simulink model "tasks_union_2"  (R2020b)
settings: Solver=FixedStepAuto  StartTime=0.0  StopTime=5  FixedStep=0.001  RelTol=1e-3
values from neighbouring files (symbols this model uses):
  a = evalin('base','a')    [Coriolis.m]    (also in init.m = 0.5)
  a0 = 0.99    [init.m]
  ac = mass_can*(l1*l2)    (= 0.5)    [init.m]
  berta = 0.98    [init.m]
  csi = 1    [init.m]
  D_high = [sqrt(4*M*K_high(1,1)) 0; 0 sqrt(4*M*K_high(2,2))]    [init.m]
  D_low = [sqrt(4*M*K_low(1,1)) 0; 0 sqrt(4*M*K_low(2,2))]    [init.m]
  e_max = 0.01    [init.m]
  F_int_max = [2;2]    [init.m]
  F_max = [2;2]    [init.m]
  g = evalin('base','g')    [Gravity.m]    (also in init.m = 9.81)
  I1 = evalin('base','I1')    [Mass.m]    (also in init.m = 1)
  I2 = evalin('base','I2')    [Mass.m]    (also in init.m = 1)
  Ic = mass_can*l2^2    (= 0.5)    [init.m]
  K_high = [F_max(1)/e_max 0; 0 (mass_can*g)/e_max]    [init.m]
  K_low = [20 0; 0 20]    [init.m]
  l1 = evalin('base','l1')    [Gravity.m]    (also in Jacobianoa_dot.m; Mass.m; cin_dir.m; init.m = 1)
  l2 = evalin('base','l2')    [Gravity.m]    (also in Jacobianoa_dot.m; Mass.m; cin_dir.m; init.m = 1)
  M = 0.1    [init.m]
  m1 = evalin('base','m1')    [Gravity.m]    (also in Mass.m; init.m = 1)
  m2 = evalin('base','m2')    [Gravity.m]    (also in Mass.m; init.m = 1)
  mass = 0.1    [init.m]
  mass_can = 0.5    [init.m]
libraries: simulink x1
(part 2 of 2)

== matlab function tasks_union_2/RR_Model_Joint_Space/MASS^-1 ==
  data: q input size=2; ddq output size=2; F_tot input double size=2; I1 parameter; I2 parameter; l1 parameter; l2 parameter; m1 parameter; m2 parameter; grasping input; Ic parameter; mass_can parameter
function ddq = fcn(q,F_tot,I1, I2, l1, l2, m1, m2, grasping, Ic, mass_can)

mc = mass_can;

B = [((l1^2)/4)*m1 + I1 + m2*(l1^2) + m2*((l2^2)/4) + m2*l1*l2*cos(q(2)) + I2, m2*(((l1*l2)/2)*cos(q(2)) + (l2^2)/4) + I2; ...
    m2*(((l1*l2)/2)*cos(q(2)) + (l2^2)/4) + I2, m2*(l2^2)/4 + I2];

% if grasping == 1
%     Bc = [mc*((l1^2) + (l2^2) +2*l1*l2*cos(q(2))) + Ic, mc*((l2^2) + l1*l2*cos(q(2))) + Ic; ...
%           mc*((l2^2) + l1*l2*cos(q(2))) + Ic, mc*(l2^2)+ Ic];
%     B = B + Bc;
% end

ddq = B\F_tot;                      % Ftot*M^-1

end

== matlab function tasks_union_2/RR_Model_Joint_Space/MATLAB Function ==
  data: F input size=2; F_ext output double size=2; q input size=2; l1 parameter; l2 parameter
function F_ext = fcn(F,q,l1, l2)


Ja = [-l1*sin(q(1)) - l2*sin(q(1)+q(2)), -l2*sin(q(1)+q(2)); ...
    l1*cos(q(1)) + l2*cos(q(1)+q(2)), l2*cos(q(1)+q(2))];

F_ext = Ja'*F;

end

== matlab function tasks_union_2/Dyrect Kinematics ==
  data: q_dot input double size=2; dz output double size=2; q input double size=2; z output double size=2; l1 parameter; l2 parameter
function [dz,z] = fcn(q_dot,q,l1, l2)

z = zeros(2,1);
z(1) = l1*cos(q(1)) + l2*cos(q(1)+q(2));
z(2) = l1*sin(q(1)) + l2*sin(q(1)+q(2));

Ja = zeros(2,2);
Ja = [-l1*sin(q(1)) - l2*sin(q(1)+q(2)), -l2*sin(q(1)+q(2)); ...
    l1*cos(q(1)) + l2*cos(q(1)+q(2)), l2*cos(q(1)+q(2))];

dz = zeros(2,1);
dz = Ja*q_dot;

end

== matlab function tasks_union_2/PLANNER3/INTERPOLATOR OF K AND D  ==
  settings: updateMethod=DISCRETE
  data: time input; K output; kx_f input; ky_f input; D output; e_max parameter; F_max parameter; M parameter; berta parameter; a0 parameter; mass parameter; csi parameter
function [K,D] = fcn(time, kx_f, ky_f, e_max, F_max,M, berta, a0, mass, csi)

persistent kx ky time_prec

if isempty(time_prec)
    time_prec = 0;
end

if isempty(kx)
   kx = F_max(1)/e_max; 
end
if isempty(ky)
   ky = F_max(2)/e_max;
end

% everytime k is increasing in accordance with stability condition
if kx_f <= kx
    kx = kx_f;
else 
    kx_i = kx;
    k_dotx = berta*(4*a0*sqrt(kx_i/mass)*(kx_i)^(3/2))/(sqrt(kx_i) + 2*a0*csi*sqrt(kx_i));
    k_tempx = kx_i + k_dotx*(time -time_prec);
    if k_tempx > kx_f
        kx = kx_f;
    else
        kx = k_tempx;
    end
end

if ky_f <= ky
    ky = ky_f;
else 
    ky_i = ky;
    k_doty = berta*(4*a0*sqrt(ky_i/mass)*(ky_i)^(3/2))/(sqrt(ky_i) + 2*a0*csi*sqrt(ky_i));
    k_tempy = ky_i + k_doty*(time -time_prec);
    if k_tempy > ky_f
        ky = ky_f;
    else
        ky = k_tempy;
    end
end
time_prec = time;

dx = sqrt(4*kx*M);
dy = sqrt(4*ky*M);

D = diag([dx,dy]);
K = diag([kx,ky]);

end
